simulink model "radiosignaloriginal"  (R2025b)
settings: Solver=FixedStepDiscrete  StartTime=0.0  StopTime=10.0  FixedStep=1e-6  RelTol=1e-3
libraries: commdigbbndpm3 x5, commrandsrc3 x5, commchan3 x1
settings Model: Creator=Nandan Prasad  LastModifiedBy=Nandan Prasad

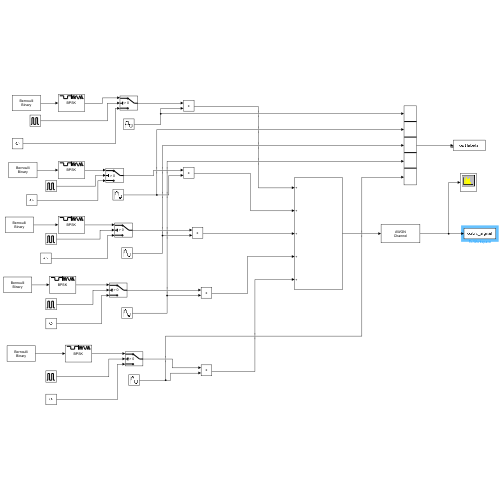
[thumbnail: Simulink's stored preview of the top-level diagram]
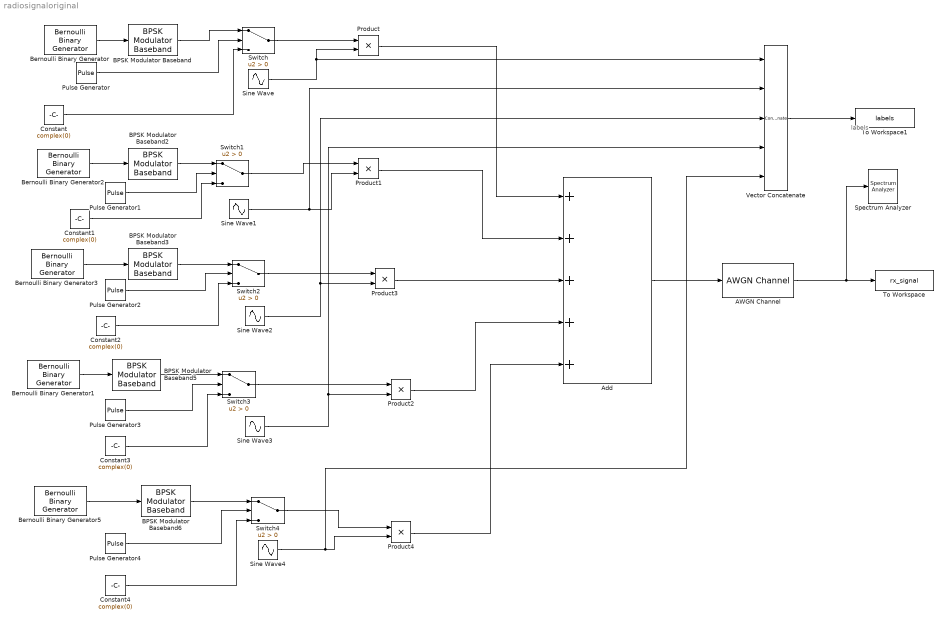
== system radiosignaloriginal ==
  note: labels
  AWGN Channel : commchan3/AWGN Channel  LegacyMode=off  NoiseMethod="Signal to noise ratio  (SNR)"  noiseMode="Signal to noise ratio  (SNR)"  EbNo=10  EsNo=10  SNR=20  BitsPerSymbol=1  SignalPower=1  SpecifySymbolPeriod=off  SamplesPerSymbol=1  SymbolPeriod=1  VarianceSource=Parameter  Variance=1  RandomStream=Global stream  Seed=67  SimulateUsing=Code generation
  Add : Sum  Inputs=+++++
  BPSK Modulator Baseband{,2..3,5..6} (5 alike) : commdigbbndpm3/BPSK Modulator Baseband  Ph=0  outDtype=double  outWordLen=16  outUDDataType=sfix(16)  outFracLenMode=Best precision  outFracLen=15  outDataTypeStr=double  outLastDataTypeStr=double
      settings: LibrarySourceBlock=|
      | commhdldigbbndpm/BPSK
      | Modulator
      | Baseband
  Bernoulli Binary Generator : commrandsrc3/Bernoulli Binary Generator  ProbabilityOfZero=0.5  SeedSource=Auto  Seed=0  SampleTime=1e-6  SamplesPerFrame=1  OutputDataType=double  SimulateUsing=Interpreted execution
  Bernoulli Binary Generator1 : commrandsrc3/Bernoulli Binary Generator  ProbabilityOfZero=0.5  SeedSource=Auto  Seed=0  SampleTime=1/1e6  SamplesPerFrame=1  OutputDataType=double  SimulateUsing=Interpreted execution
  Bernoulli Binary Generator2 : commrandsrc3/Bernoulli Binary Generator  ProbabilityOfZero=0.5  SeedSource=Auto  Seed=0  SampleTime=1/1e6  SamplesPerFrame=1  OutputDataType=double  SimulateUsing=Interpreted execution
  Bernoulli Binary Generator3 : commrandsrc3/Bernoulli Binary Generator  ProbabilityOfZero=0.5  SeedSource=Auto  Seed=0  SampleTime=1e-6  SamplesPerFrame=1  OutputDataType=double  SimulateUsing=Interpreted execution
  Bernoulli Binary Generator5 : commrandsrc3/Bernoulli Binary Generator  ProbabilityOfZero=0.5  SeedSource=Auto  Seed=0  SampleTime=1/1e6  SamplesPerFrame=1  OutputDataType=double  SimulateUsing=Interpreted execution
  Constant{,1..4} (5 alike) : Constant  Value=complex(0)  SampleTime=1e-6
  Product{,1..4} (5 alike) : Product
  Pulse Generator{,1..4} (5 alike) : DiscretePulseGenerator  PulseType=Time based  Period=10  PulseWidth=5
  Sine Wave : Sin  Frequency=2*pi*100e3  SampleTime=1e-6
  Sine Wave1 : Sin  Frequency=2*pi*200e3  SampleTime=1e-6
  Sine Wave2 : Sin  Frequency=12*pi*300e3  SampleTime=1e-6
  Sine Wave3 : Sin  Frequency=2*pi*400e3  SampleTime=1e-6
  Sine Wave4 : Sin  Frequency=2*pi*500e3  SampleTime=1e-6
  Spectrum Analyzer : SpectrumAnalyzer  WindowPosition=[599.000000,148.000000,800.000000,500.000000,]  ScopeFrameLocation=window  Method=Welch  PlotAsTwoSidedSpectrum=off  AveragingMethod=Exponential  YLimits=[-25.0192 -15.2609]
  Switch{,1..4} (5 alike) : Switch  Criteria=u2 > Threshold  SaturateOnIntegerOverflow=off  InputSameDT=off
  To Workspace : ToWorkspace  VariableName=rx_signal  SampleTime=1e-6
      settings: Save2DSignal=2-D array (concatenate along first dimension)
  To Workspace1 : ToWorkspace  VariableName=labels  SampleTime=1e-6
      settings: Save2DSignal=2-D array (concatenate along first dimension)
  Vector Concatenate : Concatenate  NumInputs=5
  wires:
  Bernoulli Binary Generator/1 -> BPSK Modulator Baseband/1
  BPSK Modulator Baseband/1 -> Switch/1
  Pulse Generator/1 -> Switch/2
  Constant/1 -> Switch/3
  Bernoulli Binary Generator2/1 -> BPSK Modulator Baseband2/1
  BPSK Modulator Baseband2/1 -> Switch1/1
  Pulse Generator1/1 -> Switch1/2
  Constant1/1 -> Switch1/3
  Bernoulli Binary Generator3/1 -> BPSK Modulator Baseband3/1
  BPSK Modulator Baseband3/1 -> Switch2/1
  Pulse Generator2/1 -> Switch2/2
  Constant2/1 -> Switch2/3
  Bernoulli Binary Generator1/1 -> BPSK Modulator Baseband5/1
  BPSK Modulator Baseband5/1 -> Switch3/1
  Pulse Generator3/1 -> Switch3/2
  Constant3/1 -> Switch3/3
  Bernoulli Binary Generator5/1 -> BPSK Modulator Baseband6/1
  BPSK Modulator Baseband6/1 -> Switch4/1
  Pulse Generator4/1 -> Switch4/2
  Constant4/1 -> Switch4/3
  Switch4/1 -> Product4/1
  Sine Wave4/1 -> Vector Concatenate/5, Product4/2
  Switch3/1 -> Product2/1
  Sine Wave3/1 -> Vector Concatenate/4, Product2/2
  Switch2/1 -> Product3/1
  Sine Wave2/1 -> Vector Concatenate/3, Product3/2
  Switch1/1 -> Product1/1
  Sine Wave1/1 -> Vector Concatenate/2, Product1/2
  Switch/1 -> Product/1
  Product/1 -> Add/1
  Product1/1 -> Add/2
  Product3/1 -> Add/3
  Product2/1 -> Add/4
  Product4/1 -> Add/5
  Add/1 -> AWGN Channel/1
  AWGN Channel/1 -> Spectrum Analyzer/1, To Workspace/1
  Sine Wave/1 -> Product/2, Vector Concatenate/1
  Vector Concatenate/1 -> To Workspace1/1
